simulink model "Main_bikesim_backup"  (R2025a)
settings: Solver=FixedStepAuto  StartTime=0.0  StopTime=inf  FixedStep=0.0005
values from neighbouring files (symbols this model uses):
  A_d = permute(A_d,[1,3,2])    [Main_sim.m]    (also in Startup_labview_v2.m; sensor_error_test_sequence.m = (eye(size(A))+Ts*A))
  Ad_t = eye(1)+Ts*A_t    [Main_sim.m]    (also in Startup_labview_v2.m = (eye(size(A_t))+Ts*A_t))
  B_d = zeros(V_n,7,1)    [Main_sim.m]    (also in Startup_labview_v2.m; sensor_error_test_sequence.m = Ts*B)
  badGPS = 0    [Main_sim.m]
  Bd_t = B_t*Ts    [Main_sim.m]    (also in Startup_labview_v2.m)
  bike_model = 1    [Main_sim.m]
  bike_params = LoadBikeParameters(bike)    [Compare_real_to_sim.m]    (also in MPC_Data_train.m = LoadBikeParameters("green"); Main_sim.m; Startup_labview_v2.m; sensor_error_test_sequence.m)
  C = mpc_outer_params.Cd    [MPC_Data_train.m]    (also in Main_sim.m = permute(C,[1,3,2]); Startup_labview_v2.m = permute(C,[1,3,2]); fromIMU2trajectory.m = (W_roll * W_roll.') / max(1, size(W_roll,2)); sensor_data_check.m = (W_roll * W_roll.') / max(1, size(W_roll,2)))
  C_t = zeros(V_n,1)    [Main_sim.m]    (also in Startup_labview_v2.m)
  counter = zeros(V_n,1)    [Main_sim.m]    (also in Startup_labview_v2.m; sensor_error_test_sequence.m = 9)
  D = mpc_outer_params.Dd    [MPC_Data_train.m]    (also in Main_sim.m = zeros(V_n,7,1); Startup_labview_v2.m = zeros(V_n,7,1))
  D_t = zeros(V_n,1)    [Main_sim.m]    (also in Startup_labview_v2.m)
  e1_max = abs(-k2*e2_max/k1)    [Startup_labview_v2.m]
  friction_coefficient = 0.004    [Main_sim.m]
  gg = 9.81    [Main_sim.m]    (also in Startup_labview_v2.m)
  hor_dis = 5    [Main_sim.m]
  I_balancing_outer = 0.0    (= 0)    [Main_sim.m]    (also in Startup_labview_v2.m; sensor_error_test_sequence.m)
  indoor = 0    [Main_sim.m]
  initial_state_estimate = initial_state    [Main_sim.m]    (also in sensor_error_test_sequence.m)
  interpolation = 0    [Main_sim.m]
  k1 = K(1)    [Startup_labview_v2.m]
  k2 = K(2)    [Startup_labview_v2.m]
  K_GPS = permute(K_GPS,[1,3,2])    [Main_sim.m]    (also in Startup_labview_v2.m)
  K_noGPS = permute(K_noGPS,[1,3,2])    [Main_sim.m]    (also in Startup_labview_v2.m)
  mpc_outer_params =     [MPC_params_train.mat]    (also in Main_sim.m = struct(); mpc_outer_params.mat)
  P_balancing_inner = 3.5    [Main_sim.m]    (also in Startup_labview_v2.m; sensor_error_test_sequence.m)
  P_balancing_outer = 3.75    [Main_sim.m]    (also in Startup_labview_v2.m; sensor_error_test_sequence.m)
  Psiref = [Psiref(1); Psiref]    [ReferenceGenerator.m]    (also in differenttest.m = [atan2(Yref(2)-Yref(1), Xref(2)-Xref(1)); differenttest_Simon.m = [psi(1); psi])
  ref_dis = 1    [Main_sim.m]    (also in differenttest.m = 0.1; differenttest_Simon.m = 0.1)
  T = [ 1,  sin(phi)*tan(th),  cos(phi)*tan(th) ... (first row only)    [Copy_of_fromIMU2trajectory.m]    (also in Main_sim.m = TransMatrix(bike_params); fromIMU2trajectory.m; sensor_error_test_sequence.m = Rz*Ry*Rx; shorttrajectory.m = table(Xref, Yref, Psiref, Vref, t, 'VariableNames', {'Xref',)
  t_ref = linspace(0, (lL-1)/Vref_test, lL)'    [differenttest.m]    (also in differenttest_Simon.m)
  Ts = 0.01    [Main_sim.m]    (also in Startup_labview_v2.m; sensor_error_test_sequence.m)
  V = round(V,1)    [Main_sim.m]    (also in Startup_labview_v2.m)
  v_init = Vref(1)    [Main_sim.m]    (also in Startup_labview_v2.m)
  Vref = zeros(length(Xref), 1)    [Refgeneration_test.m]    (also in differenttest_Simon.m = Vref_test * ones(N_line, 1))
  vv = 2    [Main_sim.m]    (also in Refgeneration.m = table_ref.v)
  Xref = [Xref;Xref2]    [ReferenceGenerator.m]    (also in concatenate.m; differenttest.m = interp1(cumulative_distance, x, equal_distances)'; differenttest_Simon.m = interp1(s, x_path, s_eq, 'linear')')
  Yref = [Yref;Yref2]    [ReferenceGenerator.m]    (also in concatenate.m; differenttest.m = interp1(cumulative_distance, y, equal_distances)'; differenttest_Simon.m = interp1(s, y_path, s_eq, 'linear')')
undefined symbols (not defined in the file or in its folder): initial_state, MPC_Ts, pert_deltadot_state, pert_deltadot_state_fun, pert_phidot_state, pert_phidot_state_fun
libraries: simulink x10, slpidlib x4, matrix_library x1, eeGeneralControl x1
(part 3 of 3)

== matlab function Main_bikesim_backup/Trajectory controller/Trajectory controller ==
  settings: updateMethod=DISCRETE  sampleTime=Ts*10
  data: closestpoint_idx input; closestpoint_heading_idx input; e1 output; e2 output; Xref_loc input; Yref_loc input; psiref_loc input; X_est input; Y_est input; psi_est input; bike_params input; v input; ref_X output; ref_Y output; ref_psi output; roll_ref output; delta_ref output; mpc_outer_params parameter; EXITFLAG output; Ad_t parameter; Bd_t parameter; C_t parameter; D_t parameter
function [e1,e2,ref_X,ref_Y,ref_psi,roll_ref,delta_ref,EXITFLAG]= fcn(closestpoint_idx, closestpoint_heading_idx,Xref_loc,Yref_loc,psiref_loc,X_est,Y_est,psi_est,bike_params,v, ...
                                                                                                             mpc_outer_params, Ad_t, Bd_t, C_t, D_t)
%% calculations on a local part of the trajectory

% Unpack parameters
g  = bike_params(1);
lr = bike_params(2);
lf = bike_params(3);
lambda = bike_params(4);

% Calculate X and Y distance from current location to selected closest
% point
dx = X_est - Xref_loc(closestpoint_idx,1);
dy = Y_est - Yref_loc(closestpoint_idx,1);

% Calculate difference in current heading and heading in reference point 
% And limit D_psiref  between -2pi and 2pi
D_psiref=psiref_loc(closestpoint_idx+1,1)-psiref_loc(closestpoint_idx,1);
if D_psiref>=pi
    D_psiref=mod(D_psiref,-2*pi);
end
if D_psiref<=-pi
    D_psiref=mod(D_psiref,2*pi);
end

if closestpoint_idx > 1
    %IMPROVEMENT: implement an interpolation algoritm
    % Calculate distence between point before closest point and current location
    dist_true_previous = sqrt((Xref_loc(closestpoint_idx-1,1)-X_est)^2+(Yref_loc(closestpoint_idx-1,1)-Y_est)^2);
    % Angle of line between previous closest point and current location
    alpha_star = atan((Yref_loc(closestpoint_idx-1,1)-Y_est)/(Xref_loc(closestpoint_idx-1,1)-X_est));
    % heading previous closest point - alpha star
    alpha_projected_dist = alpha_star-psiref_loc(closestpoint_idx,1);
    % the distance from the previous closest point to the projection of the bike on the trajectory
    Projected_dist = abs(dist_true_previous*cos(alpha_projected_dist));

    compared_dist = sqrt((Xref_loc(closestpoint_idx,1)-Xref_loc(closestpoint_idx-1,1))^2+(Yref_loc(closestpoint_idx,1)-Yref_loc(closestpoint_idx-1,1))^2);

    % If bike passes closest point, the heading of the next point will be taken
    if Projected_dist >= compared_dist
        closestpoint_heading_idx = closestpoint_idx+1;
    end
end

%calculate e1 and e2        
e1= dy*cos(psiref_loc(closestpoint_heading_idx,1)) - dx*sin(psiref_loc(closestpoint_heading_idx,1)); % this make e1 include "direction" automatically
e2= psi_est-psiref_loc(closestpoint_heading_idx,1); %calculate e2

% closest point on the local trajectory
ref_X=Xref_loc(closestpoint_idx,1);
ref_Y=Yref_loc(closestpoint_idx,1);
ref_psi=psiref_loc(closestpoint_heading_idx,1);

 % keep heading error should be between -pi 2 pi
e2 = wrapToPi(e2);
%e2=mod(e2+pi,2*pi)-pi; 

% MPC controller
A=mpc_outer_params.Ad;
B=mpc_outer_params.Bd;
C=mpc_outer_params.Cd;
D=mpc_outer_params.Dd;
N=mpc_outer_params.N;
Q=mpc_outer_params.Q;
Pf=mpc_outer_params.Pf;
R=mpc_outer_params.R;
F=mpc_outer_params.F;
G=mpc_outer_params.G;
h_mpc=mpc_outer_params.h;

x=[e1 e2]';

%Assemble the Q_bar and R_bar
Q_bar = blkdiag(kron(eye(N-1),Q),Pf);
R_bar = kron(eye(N),R);
%quadratic objective form
H=blkdiag(Q_bar,R_bar);
f=[]; %f is empty due to the lack of linear terms in cost func

%equality constraints
[rowA,colA]=size(A);
[rowB,colB]=size(B);

%Aeq1=zeros(N*rowA,N*colA);
Aeq1=kron(eye(colA),eye(N));

[rowAeq1,colAeq1]=size(Aeq1);

colAeq1Range=[1:colA:colAeq1-colA];
colAeq1Index=1;
% Todo: Replace with kron for speed 
for n=rowA:rowA:rowAeq1-rowA
    Aeq1(n+1:n+rowA,colAeq1Range(colAeq1Index):colAeq1Range(colAeq1Index)+colA-1)=-A;
    colAeq1Index=colAeq1Index+1;
end

Aeq2 = kron(eye(N),-B);

Aeq  = [Aeq1 Aeq2];
beq  = [A*x;zeros(colA*(N-1),1)];

%inequallity
Ain  = [F G];
bin  = h_mpc;

coder.extrinsic('quadprog');
coder.extrinsic('optimset');
% max time tunable...
maxTime=10;
options = optimset('Algorithm','active-set', 'Display', 'off','TolX',1e-2,'TolFun', 1e-3,'MaxTime',maxTime);

%% Optimizer

persistent Z_prev   % Z_prev is used for better guessing x0.
if isempty(Z_prev)
    Z_prev = zeros(390, 1);
end
x0 = [Z_prev(2:end); Z_prev(end)];

EXITFLAG = 0;

[Z,VN,EXITFLAG] = quadprog(2*H,f,Ain,bin,Aeq,beq,[],[],x0,options);

Z_prev = Z;

%% Building control signal

delta_ref = 0;
delta_ref=Z(colA*N+1);

if delta_ref>=pi/9
    delta_ref=pi/9;
 
end
if delta_ref<=-pi/9
    delta_ref=-pi/9;
end
eff_delta_ref = delta_ref*sin(lambda);
roll_ref = -1*atan((tan(eff_delta_ref)*(v^2/(lr+lf)))/g);
end

== matlab function Main_bikesim_backup/Trajectory controller1/Closest point finder ==
  settings: updateMethod=DISCRETE  sampleTime=Ts
  data: Xref_loc input; closestpoint_idx output; X_est input; Yref_loc input; Y_est input; closestpoint_heading_idx output
function [closestpoint_idx, closestpoint_heading_idx] = fcn(Xref_loc, X_est, Yref_loc, Y_est)
% Each referencepoint has a location (X,Y) and a heading
% The heading is defined in the startup.m file as 'the heading where its coming from' 
% Second point in local reference is current selected closest point
closestpoint_idx=2;

% Search for closest point
% Finding the closest point going forward. Stop searching once next
% distance increases

while (Xref_loc(closestpoint_idx,1)-X_est)^2 + (Yref_loc(closestpoint_idx,1)-Y_est)^2 >= (Xref_loc(closestpoint_idx+1,1)-X_est)^2+(Yref_loc(closestpoint_idx+1,1)-Y_est)^2  && closestpoint_idx <= length(Xref_loc)-2
closestpoint_idx = closestpoint_idx+1;
end

% Select same closest point (for heading error and position error)
closestpoint_heading_idx = closestpoint_idx;

== matlab function Main_bikesim_backup/Trajectory controller1/Trajectory controller ==
  settings: updateMethod=DISCRETE  sampleTime=MPC_Ts
  data: Roll_reference output; closestpoint_idx input; closestpoint_heading_idx input; Xref_loc input; Yref_loc input; psiref_loc input; X_est input; Y_est input; PSI_est input; MPC_lat_errors output; vv parameter; MPC_Ts parameter; mpc_outer_params parameter; MPC_heading_errors output; bike_params parameter; gg parameter; MPC_states output; MPC_ctrl output
function [Roll_reference, MPC_lat_errors, MPC_heading_errors, MPC_states, MPC_ctrl] = fcn(closestpoint_idx,closestpoint_heading_idx, Xref_loc, Yref_loc, psiref_loc, X_est, Y_est, PSI_est, vv, MPC_Ts, mpc_outer_params, bike_params, gg)
%% Paramater unpacking
% MPC params
A=mpc_outer_params.Ad;
B=mpc_outer_params.Bd;
C=mpc_outer_params.Cd;
D=mpc_outer_params.Dd;
N=mpc_outer_params.N;
%Q=mpc_outer_params.Q; % Q = [0.01, 0; 0, 0.01];
Q = [0.01, 0; 0, 0.01];
%Pf=mpc_outer_params.Pf; Q = [3, 0; 0, 100];
Pf = [100, 0; 0, 100];
%R=mpc_outer_params.R; R = 1
R = 1;
F=mpc_outer_params.F;
G=mpc_outer_params.G;
h_mpc=mpc_outer_params.h;

% Bike params
g  = gg;
lr = bike_params.lr;
lf = bike_params.lf;
lambda = bike_params.lambda;

%% Reference generation
[e1, e2, X_ref_interp, Y_ref_interp, PSI_ref_interp] = mpc_errors_horizon(Xref_loc, Yref_loc, X_est, Y_est, psiref_loc, PSI_est, vv, N, MPC_Ts);

% For debugging
MPC_lat_errors = e1(1:10:N);
MPC_heading_errors = e2(1:10:N);

%% Quadratic problem formulatiom

% Cost matrices
Q_bar = blkdiag(kron(eye(N-1),Q),Pf);
R_bar = kron(eye(N),R);
H = blkdiag(Q_bar,R_bar);

e_ref = reshape([e1(:), e2(:)]', [], 1);
u_ref = zeros(length(R_bar), 1);
x_ref = [e_ref; u_ref];
%f = [];
f = 2*x_ref'*H;

% Equality constraints
[rowA,colA] = size(A);

Main_Diag = eye(N * rowA);
Lower_Diag = kron(diag(ones(N-1, 1), -1), -A);
Aeq1 = Main_Diag + Lower_Diag;

Aeq2 = kron(eye(N),-B);
Aeq  = [Aeq1, Aeq2];

beq  = [A*[0;0]; zeros(colA*(N-1),1)];

% Inequallity constraints
Ain  = [F, G];
bin  = h_mpc;

coder.extrinsic('quadprog');
coder.extrinsic('optimset');
maxTime=10;
options = optimset('Algorithm','active-set', 'Display', 'off','TolX',1e-2,'TolFun', 1e-3,'MaxTime',maxTime);

%% Optimizer

persistent Z_prev   % Z_prev is used for better guessing x0.
if isempty(Z_prev)
    Z_prev = zeros(length(H), 1);
end
x0 = [Z_prev(2:end); Z_prev(end)];

EXITFLAG = 0;

[Z,VN,EXITFLAG] = quadprog(2*H,f,Ain,bin,Aeq,beq,[],[],x0,options);

Z_prev = Z;

%% Control signal

delta_ref=Z(colA*N+1);
eff_delta_ref = delta_ref*sin(lambda);

Roll_reference = 0;
Roll_reference = -1*atan((tan(eff_delta_ref)*(vv^2/(lr+lf)))/g);

%% Extract trajectory to plot MPC simulated states

MPC_states = zeros(N*rowA, 1);
MPC_ctrl = zeros(N, 1);

save_MPC_optmized = 1;
if save_MPC_optmized == 1
    MPC_states = Z(1:N*rowA);
    MPC_ctrl = Z(N*rowA+1:N*rowA+N);
end


end

function [lat_error_horizon, heading_error_horizon, X_ref_interp, Y_ref_interp, PSI_ref_interp] = mpc_errors_horizon(X_loc, Y_loc, X_est, Y_est, PSI_loc, PSI_est, vv, N, MPC_Ts)
   
    %% 1. Find the closest point on the track (Perpendicular projection approximation)
    % Calculate distance from vehicle to all track points
    dists = sqrt((X_loc(1:3) - X_est).^2 + (Y_loc(1:3) - Y_est).^2);
    [~, min_idx] = min(dists);
    
    %% 2. Calculate Arc Length (Distance along the track)
    % We need this to interpolate correctly based on speed
    % Compute distances between consecutive track points
    dX = diff(X_loc);
    dY = diff(Y_loc);
    segment_lengths = sqrt(dX.^2 + dY.^2);
    
    % Cumulative distance (Arc Length s)
    % Prepend 0 for the first point
    s_track = [0, cumsum(segment_lengths)']; 
    
    %% 3. Generate Target Arc Lengths for the Horizon
    % Start exactly at the arc length of the closest point found above
    current_s = s_track(min_idx);
    
    % Create a vector of desired distances: s, s+vT, s+2vT...
    % We generate N points
    steps = (0:N-1) * (vv * MPC_Ts);
    target_s = current_s + steps;
    
    %% 4. Interpolate Global Reference Points
    % Use linear interpolation
    X_ref_interp = interp1(s_track, X_loc, target_s, 'linear', 'extrap');
    Y_ref_interp = interp1(s_track, Y_loc, target_s, 'linear', 'extrap');
    PSI_ref_interp = interp1(s_track, PSI_loc, target_s, 'linear', 'extrap');

    %% 7. Heading error
    heading_error_horizon = PSI_est - PSI_ref_interp;

    %% 6. Lateral error
    dx = X_est - X_ref_interp;
    dy = Y_est - Y_ref_interp;
   
    c = cos(PSI_est);
    s = sin(PSI_est);
    
    % y_error is lateral error over the defined horizon
    lat_error_horizon = -s .* dx + c .* dy;
    
end

== matlab function Main_bikesim_backup/Unstable bike model1/Nonlinear Bicycle model/MATLAB Function ==
  data: States input; xdot output; Steering_rate input; Speed input; disturbances input; bike_params input
function xdot  = fcn(States, Steering_rate, Speed, disturbances, bike_params)
% Unpacked bike_params
    g = bike_params(1);
    h = bike_params(2);
    lr = bike_params(3);
    lf = bike_params(4);
    lambda = bike_params(5);
    c = bike_params(6);
    %m = bike_params(7);
    %h_imu = bike_params(8);

phi =   States(1);%roll

%% debug
phi_max = deg2rad(20);   % something reasonable
phi = max(min(phi, phi_max), -phi_max);
%%

delta = States(2);%steering angle
phi_d = States(3);%rollrate


% xdot = [phidot deltadot phiddot]
xdot1 = phi_d + disturbances(1);
xdot2 = Steering_rate + disturbances(2);
xdot3 = (g/h)*sin(phi) + ((lr*Speed)/((lr+lf)*h))/(cos(sin(lambda)*delta)^2)*sin(lambda)*Steering_rate ...
                                  + ((Speed^2/h)-(g*lr*c/(h^2*(lr+lf))))*sin(lambda)*tan(delta);

% linearized
% xdot3 = (g/h)*phi + ((lr*Speed)/((lr+lf)*h))*Steering_rate + ((Speed^2/h)-(g*lr*c/(h^2*(lr+lf))))*sin(lambda)*delta;

xdot = [xdot1 xdot2 xdot3]';

== matlab function Main_bikesim_backup/Trajectory controller1/MATLAB Function ==
  data: u input; mpc_sim_e1 output; mpc_sim_e2 output
function [mpc_sim_e1, mpc_sim_e2] = fcn(u)

mpc_sim_e1 = u(1:20:130*2 - 1);
mpc_sim_e2 = u(2:20:130*2);

== matlab function Main_bikesim_backup/Unstable bike model1/Track bycicle pose, poistion and direction/Derivative of positions ==
  data: Speed input; beta input; psi input; Xdot output; Ydot output
function [Xdot, Ydot]  = fcn(Speed, beta, psi)

Xdot = Speed * cos(psi + beta);
Ydot = Speed * sin(psi + beta);

== matlab function Main_bikesim_backup/Unstable bike model1/Track bycicle pose, poistion and direction/MATLAB Function ==
  data: Speed input; steer_angle input; beta output; bike_params input; psi_dot output
function [beta, psi_dot] = fcn(Speed, steer_angle, bike_params)
lr       = bike_params(1);
lf       = bike_params(2);
lambda  = bike_params(3);

eff_steering = steer_angle*sin(lambda);

beta = atan(lr /(lr+lf) * tan(eff_steering) );
psi_dot = (Speed / lr) * sin(beta);

== matlab function Main_bikesim_backup/Selection of local reference from total reference1/Local reference selection & stop funcion ==
  data: last_ids input; ids output; xref input; local_Xref output size=Nn [..30000]; local_Yref output size=Nn [..30000]; local_Psiref output size=Nn [..30000]; local_Vref output size=Nn; local_tref output size=Nn; yref input; psiref input; Vref input; closest_point input; tref input; ref_dis parameter; hor_dis parameter; stop output; abort input; est input
function [ids,local_Xref,local_Yref,local_Psiref,local_Vref,local_tref,stop] = fcn(last_ids,xref,yref,psiref,Vref, closest_point, tref, ref_dis, hor_dis,abort,est)
% Local reference trajectory starts at point before the current closest
% point and has a length of M
ids=last_ids+closest_point-2;      % calculate the initial index of the points that will be sent to next block (first point of local_ref)

Ns=ceil(hor_dis/ref_dis);          % hor_dis, ref_dis are definited in "StudentProject2021.m", Ns is the length of the local trajectory sent to next block
M=ids+Ns;                          % calculate the end index of the local reference
n=size(xref,1);                    % length of whole trajectory  

if M>n                             % if reached near end of reference, local trajectry becomes shorter
    M=n;
    %disp('Bike position close to end of reference so that local reference partly beyoined the reference.'); 
end

% Temporary simulation STOP to prevent singularity error once approaching
% the end of the trajectory
% Simulation stops before the end of the reference trajectory
stop = 0;
if ids >= n-ceil(n/20)
    stop = 1;
    disp('Bike close to end of trajectory.');
end


% Start always at second value of total reference
if ids<2
ids = 2;
end

% Select local reference from total reference
local_Xref = xref(ids-1:M,1);
local_Yref = yref(ids-1:M,1);
local_Psiref = psiref(ids-1:M,1);
local_tref = tref(ids-1:M,1);
local_Vref = Vref(ids-1:M,1);


% If an abort is issued, the bike aborts the pre-defined reference and
% follow the abort-reference instead
if(abort)
    [local_Xref,local_Yref,local_Psiref] = genAbortTraj(est(1),est(2),est(3),Ns);
end

end


function [x_ref,y_ref,psi_ref] = genAbortTraj(x_est,y_est,psi_est,N)


step = 0.1; %Step size
r  = 5;
%N = 50;

x_ref = zeros(N,1);
y_ref = zeros(N,1);
psi_ref = zeros(N,1);
x_ref(1) = x_est;
y_ref(1) = y_est;
psi_ref(1) = psi_est;

% CALCULATE CENTER OF CIRCLE 
offset_x = r * sin(-psi_est);
offset_y = r * cos(-psi_est);
x_center = x_est + offset_x;
y_center = y_est + offset_y;

i = 1;
for t = step:step:(N*step-1)
    i = i+1;
    x_ref(i) = r*sin(-t+pi-psi_est) + x_center;
    y_ref(i) = r*cos(-t+pi-psi_est) + y_center;
    psi_ref(i) = atan2(y_ref(i)-y_ref(i-1),x_ref(i)-x_ref(i-1));  
end

end
